simulink model "Subsystem11"  (R2020b)
settings: Solver=VariableStepAuto  StartTime=0.0  StopTime=0.4  RelTol=1e-3
model workspace (MAT data in the model file):
  Kd = Simulink.Parameter
  Kd.Value = 0.48976
  Kd.DataType = 'auto'
  Kd.Dimensions = [1 1]
  Ki = Simulink.Parameter
  Ki.Value = 4810.143
  Ki.DataType = 'auto'
  Ki.Dimensions = [1 1]
  Kp = Simulink.Parameter
  Kp.Value = 97.11
  Kp.DataType = 'auto'
  Kp.Dimensions = [1 1]
  N = Simulink.Parameter
  N.Value = 100000
  N.DataType = 'auto'
  N.Dimensions = [1 1]
settings Model: DataDictionary=motor.sldd  Creator=sushma  LastModifiedBy=sushma
settings DataIOCC: SaveOutput=off  SaveTime=off

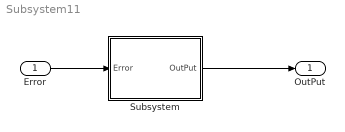
== system Subsystem11 ==
  Error : Inport  OutDataTypeStr=double  PortDimensions=1  SampleTime=0
  Subsystem : Subsystem  TreatAsAtomicUnit=on
  OutPut : Outport  OutDataTypeStr=double  PortDimensions=1  SampleTime=0
  wires:
  Error/1 -> Subsystem/1(Error)
  Subsystem/1(OutPut) -> OutPut/1

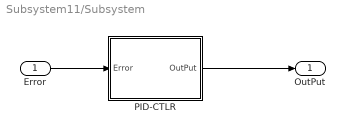
== system Subsystem11/Subsystem ==
  Error : Inport
  PID-CTLR : Subsystem
  OutPut : Outport
  wires:
  Error/1 -> PID-CTLR/1(Error)
  PID-CTLR/1(OutPut) -> OutPut/1

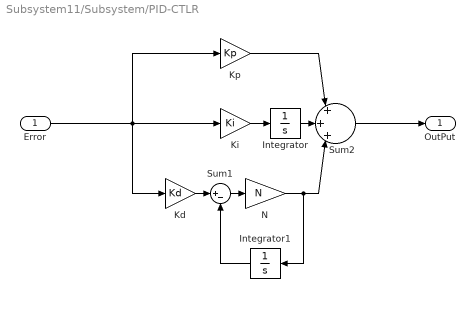
== system Subsystem11/Subsystem/PID-CTLR ==
  Error : Inport  OutDataTypeStr=double  PortDimensions=1  SampleTime=0
  Integrator : Integrator
  Integrator1 : Integrator
  Kd : Gain  Gain=Kd
  Ki : Gain  Gain=Ki
  Kp : Gain  Gain=Kp
  N : Gain  Gain=N
  Sum1 : Sum  Inputs=|+-
  Sum2 : Sum  Inputs=|+|+|+|
  OutPut : Outport  OutDataTypeStr=double  PortDimensions=1  SampleTime=0
  wires:
  Sum1/1 -> N/1
  Kd/1 -> Sum1/1
  Error/1 -> Ki/1, Kp/1, Kd/1
  Kp/1 -> Sum2/1
  Integrator/1 -> Sum2/2
  Integrator1/1 -> Sum1/2
  N/1 -> Integrator1/1, Sum2/3
  Sum2/1 -> OutPut/1
  Ki/1 -> Integrator/1
